simulink library "WBToolboxLibrary"  (R2014b)
settings: Solver=ode45  StartTime=0.0  StopTime=10.0  RelTol=1e-3
undefined symbols (not defined in the file): WBT_modelName, WBT_robotName, WBT_wbiFilename, WBT_wbiList
libraries: simulink x1
(part 1 of 2)
settings Model: Creator=jorhabib  LastModifiedBy=makaveli

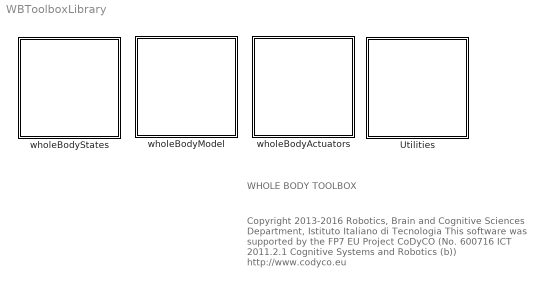
== system WBToolboxLibrary ==
  note: WHOLE BODY TOOLBOX
  note: Copyright  2013-2016 Robotics, Brain and Cognitive Sciences Department, Istituto Italiano di Tecnologia
      | This software was supported by the FP7 EU Project CoDyCO (No. 600716 ICT 2011.2.1 Cognitive Systems and Robotics (b))
      | http://www.codyco.eu
  Utilities : Subsystem
      mask Display: image(imread('utilities.png'))
  wholeBodyActuators : Subsystem
      mask Display: image(imread('wholeBodyActuators.png'),'center')
  wholeBodyModel : Subsystem
      mask Display: image(imread('wholeBodyModel.png'),'center')
  wholeBodyStates : Subsystem
      mask Display: image(imread('wholeBodyStates.png'),'center');

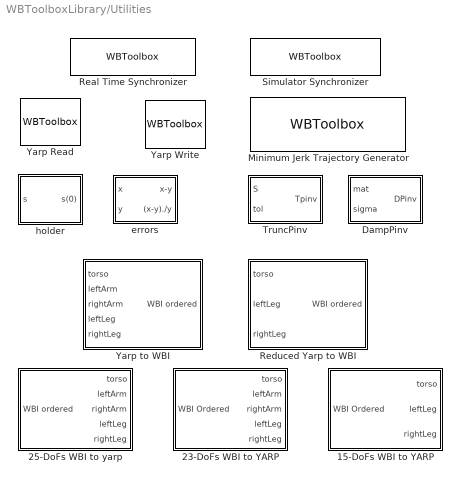
== system WBToolboxLibrary/Utilities ==
  15-DoFs WBI to YARP : Subsystem
      mask help: This is a 23-DoF iCub specific block that swaps first and third joints of the iCub torso from a WBI whole body state reading.
  23-DoFs WBI to YARP : Subsystem
      mask help: This is a 23-DoF iCub specific block that swaps first and third joints of the iCub torso from a WBI whole body state reading.
  25-DoFs WBI to yarp : Subsystem  mask(WBI to YARP){}
      mask help: This is a 25-DOF iCub specific block that swaps first and third joints of the iCub torso from a WBI whole body state reading.
  DampPinv : Subsystem  mask{tol=1e-4}
      mask prompts: tol "Tolerance"
  Minimum Jerk Trajectory Generator : S-Function  FunctionName=WBToolbox  Parameters='MinimumJerkTrajectoryGenerator',sampleTime, settlingTime, firstDerivatives, secondDerivatives, explicitInitialValue, externalSettlingTime  SFunctionDeploymentMode=off  EnableBusSupport=off  mask(Minimum Jerk Trajectory Generator){externalSettlingTime=off, settlingTime=3, sampleTime=0.01, firstDerivatives=on, secondDerivatives=on, explicitInitialValue=off}
      mask prompts: externalSettlingTime "External Settling Time"; settlingTime "Settling Time"; sampleTime "Sample Time"; firstDerivatives "Output First Derivative"; secondDerivatives "Output Second Derivative"; explicitInitialValue "Explicit Initial Value"
      mask help:
      | This block wraps the minJerkTrajGen class from iCub::ctrl::minJerkTrajGen.
      |
      | The Minimum Jerk Trajectory Generator is approximated using a
      | 3rd order LTI dynamical system
      | (for more details see [1]).
      | Position, velocity and acceleration trajectories are computed.
      |  The main advantage with respect to the standard polynomial
      | form is that if the reference value yd changes
      | there is no need to recompute the filter coefficients.
      |
      | [1] Pattacini, U.; Nori, F.; Natale, L.; Metta, G.; Sandini, G., "An experimental evaluation of a novel minimum-jerk cartesian controller for humanoid robots," in Intelligent Robots and Systems (IROS), 2010 IEEE/RSJ International Conference on , vol., no., pp.1668-1674, 18-22 Oct. 2010
      | doi: 10.1109/IROS.2010.5650851
      | URL: http://ieeexplore.ieee.org/stamp/stamp.jsp?tp=&arnumber=5650851&isnumber=5648787
      mask Callback externalSettlingTime:
      | externalSettlingTime = get_param(gcb, 'externalSettlingTime');
      | visibility = get_param(gcb, 'MaskVisibilities');
      | if(strcmp(externalSettlingTime, 'on'))
      |     visibility{2} = 'off';
      | else
      |     visibility{2} = 'on';
      | end
      | set_param(gcb, 'MaskVisibilities',visibility);
      | clear externalSettlingTime
      mask Display:
      | firstDer = get_param(gcb, 'firstDerivatives');
      | secondDer = get_param(gcb, 'secondDerivatives');
      | initialValues = get_param(gcb, 'explicitInitialValue');
      | externalSettlingTimeParam = get_param(gcb, 'externalSettlingTime');
      | 
      | %Inputs
      | portIndex = 2;
      | port_label('input', 1, 'Reference')
      | if(strcmp(initialValues, 'on'))
      |     port_label('input', portIndex, 'Initial Value')
      |     portIndex = portIndex + 1;
      | end
      | 
      | if(strcmp(externalSettlingTimeParam, 'on'))
      |     port_label('input', portIndex, 'Settling Time')
      |     portIndex = portIndex + 1;
      | end
      | 
      | %Outputs
      | port_label('output', 1, 'Signal')
      | secondDerPortIndex = 2;
      | if(strcmp(firstDer, 'on'))
      |     port_label('output', 2, 'First Derivative')
      |     secondDerPortIndex = secondDerPortIndex + 1;
      | end
      | if(strcmp(secondDer, 'on'))
      |     port_label('output', secondDerPortIndex, 'Second Derivative')
      | end
  Real Time Synchronizer : S-Function  FunctionName=WBToolbox  Parameters='RealTimeSynchronizer',period  SFunctionDeploymentMode=off  EnableBusSupport=off  mask(Real Time Synchronizer){period=0.01}
      mask prompts: period "Controller Period (in seconds)"
      mask help:
      | This block slows down the simulation trying to match the period specified
      | as parameter (in seconds).
      | The bigger the period the more probable
      | is that Simulink can remain synched with it.
      mask Display: disp('Real Time Synchronizer')
  Reduced Yarp to WBI : Subsystem  mask(YARP to wbi){}
      mask help:
      | DEPRECATED
      |
      | Please use the explicit 25-DOF or the 23-DOF utility.
      | This block will soon be removed from the Library
      |
      | This is a 25-DOF iCub specific block which swaps the readings of the first and third joint of the torso to comply with WBI order.
  Simulator Synchronizer : S-Function  FunctionName=WBToolbox  Parameters='SimulatorSynchronizer',period, serverPortName, clientPortName  SFunctionDeploymentMode=off  EnableBusSupport=off  mask(Simulator Synchronizer){period=0.01, serverPortName='/clock/rpc', clientPortName='/WBT_synchronizer/rpc:o'}
      mask prompts: period "Controller Period (in seconds)"; serverPortName "Server Port Name"; clientPortName "Client Port Name"
      mask help:
      | This block synchronizes with the external simulation on a simulator
      | (only Gazebo is supported at the moment).
      mask Display: disp('Simulator Synchronizer')
  TruncPinv : Subsystem  mask{tol=1e-4}
      mask prompts: tol "Tolerance"
  Yarp Read : S-Function  FunctionName=WBToolbox  Parameters='YarpRead',portName,signalSize,blocking,timestamp,autoconnect,errorOnConnection  SFunctionDeploymentMode=off  EnableBusSupport=off  mask(YARP Read){portName='/portname', signalSize=1, blocking=off, timestamp=on, autoconnect=on, errorOnConnection=on}
      mask prompts: portName "Source Port Name"; signalSize "Port Size"; blocking "Blocking Read"; timestamp "Read Timestamp"; errorOnConnection "Error on missing connection"
      mask help:
      | This block behaves as the command 'yarp read'.
      | By default it has the option 'Autoconnect' active, which means that the user
      | can only specify the name of the port ('Source Port Name') from which readings are desired,
      | along with the size of the expected data (e.g. 3 when reading the torso state).
      | When the user unchecks 'Autoconnect' 'Opened Port Name' field shows up
      | corresponding to the name of the port the block will create
      | but won't connect to anything.
      | At this point the output will be always zero, until the user connects it
      | to some other port from command line by issuing 'yarp connect [from] [dest]'.
      | In this case an additional output, called 'signal' will be added which will output
      | 1 if the port has received at least one data, or 0 otherwise.
      mask Callback autoconnect:
      | autoconnect_val = get_param(gcb, 'Autoconnect');
      | prompt_string = get_param(gcb, 'MaskPrompts');
      | if(strcmp(autoconnect_val, 'on'))
      |     prompt_string{1} = 'Source Port Name';
      |     set_param(gcb, 'MaskVisibilities',{'on';'on';'on';'on';'on';'on'});
      | else
      |     prompt_string{1} = 'Opened Port Name';
      |     set_param(gcb, 'MaskVisibilities',{'on';'on';'on';'on';'on';'off'});
      | end
      | set_param(gcb, 'MaskPrompts', prompt_string);
      | clear autoconnect_val prompt_string
      mask Display:
      | port_label('output', 1, 'signal');
      | portNumber = 1;
      | if (timestamp)
      |     portNumber = portNumber + 1;
      |     port_label('output', portNumber, 'timestamp');
      | end
      | 
      | if (~autoconnect)
      |     portNumber = portNumber + 1;
      |     port_label('output', portNumber, 'status');
      | end
  Yarp Write : S-Function  FunctionName=WBToolbox  Parameters='YarpWrite',portName,autoconnect,errorOnConnection  SFunctionDeploymentMode=off  EnableBusSupport=off  mask(YARP Write){portName='/portname', autoconnect=off, errorOnConnection=on}
      mask prompts: portName "Opened Port Name"; errorOnConnection "Error on missing connection"
      mask help:
      | This block behaves as the command 'yarp write'.
      |
      | By default this block opens a port names as the "Opened Port Name" parameter
      | and stream the input signal to that port.
      | If the option "Autoconnect" is specified, the first parameter become the
      | name of the target port to which the data will be stramed,
      | e.g. like "yarp write ... /destinationPort"
      mask Callback autoconnect:
      | autoconnect_val = get_param(gcb, 'Autoconnect');
      | prompt_string = get_param(gcb, 'MaskPrompts');
      | if(strcmp(autoconnect_val, 'on'))
      |     prompt_string{1} = 'Destination Port Name';
      |     set_param(gcb, 'MaskVisibilities',{'on';'on';'on'});
      | else
      |     prompt_string{1} = 'Opened Port Name';
      |     set_param(gcb, 'MaskVisibilities',{'on';'on';'off'});
      | end
      | set_param(gcb, 'MaskPrompts', prompt_string);
      | clear autoconnect_val prompt_string
      mask Display: disp('Yarp Write')
  Yarp to WBI : Subsystem  mask(YARP to wbi){}
      mask help:
      | DEPRECATED
      |
      | Please use the explicit 25-DOF or the 23-DOF utility.
      | This block will soon be removed from the Library
      |
      | This is a 25-DOF iCub specific block which swaps the readings of the first and third joint of the torso to comply with WBI order.
  errors : Subsystem  mask(Errors){}
      mask help:
      | Computes two kinds of errors. The first is just the difference between x
      | and y while the second is the ratio (x-y)/y.
  "holder " : Subsystem  mask(Holder){}
      mask help: This block holds the first input value during the simulation.

== system WBToolboxLibrary/wholeBodyActuators ==
  Set LowLevel PIDs : Subsystem  InitFcn=|  mask(Set Low Level PIDs){pidParameters='', pidType=Torque, robotName=WBT_robotName, localName=WBT_modelName, wbiFile=WBT_wbiFilename, wbiList=WBT_wbiList}
      | if ~exist('WBT_robotName','var')
      |     WBT_robotName = '';
      | end
      | if ~exist('WBT_modelName','var')
      |     WBT_modelName = 'WBT_simulink';
      | end
      | if ~exist('WBT_wbiFilename','var')
      |     WBT_wbiFilename = 'yarpWholeBodyInterface.ini';
      | end
      | if ~exist('WBT_wbiList','var')
      |     WBT_wbiList = 'ROBOT_TORQUE_CONTROL_JOINTS';
      | end
      mask prompts: pidParameters "PID parameter"; pidType "PID Type"; robotName "Robot Port Name"; localName "Model Name"; wbiFile "WBI filename"; wbiList "WBI list name"
      mask help:
      | This block sets the low level PID values for the robot actuators.
      |
      | If only one gain file is specified, those gains are loaded at startup.
      | Otherwise an additional port to this block is added which accept an integer
      | representing the index in the list of gains to be loaded (also at runtime)
      |
      | Assuming DoFs is the number of degrees of freedom of the robot,
      | Parameters:
      | - PID Parameter: String specifying either a file containing the PIDs for the
      |                  low level control, or a list of files (in yarp Bottle format).
      |
      | - Robot Port Name: Name of the ports opened by the robot. (e.g. icub).
      |                    Set an empty string ('') to use the name specified in the
      |                    Whole Body Interface configuration file.
      | - Model Name: Prefix name of the ports opened by the underlying Whole Body Interface.
      | - WBI filename: name of the file containing the configuration of the Whole Body Interface
      | - WBI List Name: name of the list of joints used to configure the Whole Body Interface
      mask TypeOptions pidType: Position | Torque
      mask Callback pidType:
      | % Get the mask parameter values. This is a cell
      | %   array of strings.
      | maskStr = get_param(gcb,'pidType');
      | if strcmp(maskStr, 'Position')
      |     set_param(gcb,'BackgroundColor', '[0.5137, 0.8510, 0.6706, 1.0]');
      | elseif strcmp(maskStr, 'Position Direct')
      |     set_param(gcb,'BackgroundColor', '[0.3922, 0.7882, 0.3451, 1.0]');
      | elseif strcmp(maskStr, 'Velocity')
      |     set_param(gcb,'BackgroundColor', '[0.5137, 0.6745, 1.0000, 1.0]');
      | elseif strcmp(maskStr, 'Torque')
      |     set_param(gcb,'BackgroundColor', '[0.8275, 0.5765, 0.6039, 1.0]');
      | end
      | clear  maskStr
      mask Display:
      | pidType = get_param(gcb,'pidType');
      | description = sprintf('Set Low Level\n%s PIDs', pidType);
      | disp(description);
  Set References : Subsystem  InitFcn=|  mask(Set References){controlType=Position, robotName=WBT_robotName, localName=WBT_modelName, wbiFile=WBT_wbiFilename, wbiList=WBT_wbiList}
      | if ~exist('WBT_robotName','var')
      |     WBT_robotName = '';
      | end
      | if ~exist('WBT_modelName','var')
      |     WBT_modelName = 'WBT_simulink';
      | end
      | if ~exist('WBT_wbiFilename','var')
      |     WBT_wbiFilename = 'yarpWholeBodyInterface.ini';
      | end
      | if ~exist('WBT_wbiList','var')
      |     WBT_wbiList = 'ROBOT_TORQUE_CONTROL_JOINTS';
      | end
      mask prompts: controlType "Control Mode"; robotName "Robot Port Name"; localName "Model Name"; wbiFile "WBI filename"; wbiList "WBI list name"
      mask help:
      | This block sets the references for the robot actuators.
      | The type of control mode is specified as a parameter in the block.
      |
      | Assuming DoFs is the number of degrees of freedom of the robot,
      | Input:
      | - References: Vector of size DoFs, representing the references to be sent
      |                 to the robot controlled joints.
      |
      | Parameters:
      | - Control Mode: The control mode. Choose one of the supplied mode.
      |
      | - Robot Port Name: Name of the ports opened by the robot. (e.g. icub).
      |                    Set an empty string ('') to use the name specified in the
      |                    Whole Body Interface configuration file.
      | - Model Name: Prefix name of the ports opened by the underlying Whole Body Interface.
      | - WBI filename: name of the file containing the configuration of the Whole Body Interface
      | - WBI List Name: name of the list of joints used to configure the Whole Body Interface
      mask TypeOptions controlType: Position | Position Direct | Velocity | Torque | Open Loop
      mask Callback controlType:
      | % Get the mask parameter values. This is a cell
      | %   array of strings.
      | maskStr = get_param(gcb,'controlType');
      | if strcmp(maskStr, 'Position')
      |     set_param(gcb,'BackgroundColor', '[0.5137, 0.8510, 0.6706, 1.0]');
      | elseif strcmp(maskStr, 'Position Direct')
      |     set_param(gcb,'BackgroundColor', '[0.3922, 0.7882, 0.3451, 1.0]');
      | elseif strcmp(maskStr, 'Velocity')
      |     set_param(gcb,'BackgroundColor', '[0.5137, 0.6745, 1.0000, 1.0]');
      | elseif strcmp(maskStr, 'Torque')
      |     set_param(gcb,'BackgroundColor', '[0.8275, 0.5765, 0.6039, 1.0]');
      | elseif strcmp(maskStr, 'Open Loop')
      |     set_param(gcb,'BackgroundColor', '[0.98, 0.98, 0.98, 1.0]');
      | end
      | clear  maskStr
      mask Display:
      | disp(get_param(gcb,'controlType'))
      | %port_label('input',1,'References')

== system WBToolboxLibrary/wholeBodyModel ==
  Dynamics : Subsystem
      mask Display: image(imread('Dynamics.png'))
  Jacobians : Subsystem
      mask Display: image(imread('jacobian.png'))
  Kinematics : Subsystem
      mask Display: image(imread('forwardKinematics.png'))

== system WBToolboxLibrary/wholeBodyStates ==
  Get Estimate : Subsystem  InitFcn=|  mask(Get Estimate){estimateType=Joints Position, robotName=WBT_robotName, localName=WBT_modelName, wbiFile=WBT_wbiFilename, wbiList=WBT_wbiList}
      | if ~exist('WBT_robotName','var')
      |     WBT_robotName = '';
      | end
      | if ~exist('WBT_modelName','var')
      |     WBT_modelName = 'WBT_simulink';
      | end
      | if ~exist('WBT_wbiFilename','var')
      |     WBT_wbiFilename = 'yarpWholeBodyInterface.ini';
      | end
      | if ~exist('WBT_wbiList','var')
      |     WBT_wbiList = 'ROBOT_TORQUE_CONTROL_JOINTS';
      | end
      mask prompts: estimateType "Estimate Type"; robotName "Robot Port Name"; localName "Model Name"; wbiFile "WBI filename"; wbiList "WBI list name"
      mask help:
      | This block get the estimate of the specified type
      |
      | Assuming DoFs is the number of degrees of freedom of the robot,
      | Output:
      | - References: Vector of size DoFs, representing the estimate requested.
      |
      | Parameters:
      | - Control Mode: The control mode. Choose one of the supplied mode.
      |
      | - Robot Port Name: Name of the ports opened by the robot. (e.g. icub).
      |                    Set an empty string ('') to use the name specified in the
      |                    Whole Body Interface configuration file.
      | - Model Name: Prefix name of the ports opened by the underlying Whole Body Interface.
      | - WBI filename: name of the file containing the configuration of the Whole Body Interface
      | - WBI List Name: name of the list of joints used to configure the Whole Body Interface
      mask TypeOptions estimateType: Joints Position | Joints Velocity | Joints Acceleration | Joints Torque
      mask Callback estimateType:
      | % Get the mask parameter values. This is a cell
      | %   array of strings.
      | 
      | maskStr = get_param(gcb,'estimateType');
      | if strcmp(maskStr, 'Joints Position')
      |     set_param(gcb,'BackgroundColor', '[0.5137, 0.8510, 0.6706, 1.0]');
      | elseif strcmp(maskStr, 'Joints Velocity')
      |     set_param(gcb,'BackgroundColor', '[0.5137, 0.6745, 1.0000, 1.0]');
      | elseif strcmp(maskStr, 'Joints Acceleration')
      |     set_param(gcb,'BackgroundColor', '[0.9255, 0.8706, 0.1333, 1.0]');
      | elseif strcmp(maskStr, 'Joints Torque')
      |     set_param(gcb,'BackgroundColor', '[0.8275, 0.5765, 0.6039, 1.0]');
      | end
      | clear  maskStr
      mask Display:
      | %disp(get_param(gcb,'estimateType'))
      | port_label('output',1,get_param(gcb,'estimateType'))
  Get Limits : Subsystem  InitFcn=|  mask(Get Estimate){limitsType=Position, robotName=WBT_robotName, localName=WBT_modelName, wbiFile=WBT_wbiFilename, wbiList=WBT_wbiList}
      | if ~exist('WBT_robotName','var')
      |     WBT_robotName = '';
      | end
      | if ~exist('WBT_modelName','var')
      |     WBT_modelName = 'WBT_simulink';
      | end
      | if ~exist('WBT_wbiFilename','var')
      |     WBT_wbiFilename = 'yarpWholeBodyInterface.ini';
      | end
      | if ~exist('WBT_wbiList','var')
      |     WBT_wbiList = 'ROBOT_TORQUE_CONTROL_JOINTS';
      | end
      mask prompts: limitsType "Limits Type"; robotName "Robot Port Name"; localName "Model Name"; wbiFile "WBI filename"; wbiList "WBI list name"
      mask help:
      | This block get the estimate of the specified type
      |
      | Assuming DoFs is the number of degrees of freedom of the robot,
      | Output:
      | - References: Vector of size DoFs, representing the estimate requested.
      |
      | Parameters:
      | - Control Mode: The control mode. Choose one of the supplied mode.
      |
      | - Robot Port Name: Name of the ports opened by the robot. (e.g. icub).
      |                    Set an empty string ('') to use the name specified in the
      |                    Whole Body Interface configuration file.
      | - Model Name: Prefix name of the ports opened by the underlying Whole Body Interface.
      | - WBI filename: name of the file containing the configuration of the Whole Body Interface
      | - WBI List Name: name of the list of joints used to configure the Whole Body Interface
      mask TypeOptions limitsType: Position
      mask Callback limitsType:
      | % Get the mask parameter values. This is a cell
      | %   array of strings.
      | 
      | maskStr = get_param(gcb,'limitsType');
      | if strcmp(maskStr, 'Joints Position')
      |     set_param(gcb,'BackgroundColor', '[0.5137, 0.8510, 0.6706, 1.0]');
      | elseif strcmp(maskStr, 'Joints Velocity')
      |     set_param(gcb,'BackgroundColor', '[0.5137, 0.6745, 1.0000, 1.0]');
      | elseif strcmp(maskStr, 'Joints Acceleration')
      |     set_param(gcb,'BackgroundColor', '[0.9255, 0.8706, 0.1333, 1.0]');
      | elseif strcmp(maskStr, 'Joints Torque')
      |     set_param(gcb,'BackgroundColor', '[0.8275, 0.5765, 0.6039, 1.0]');
      | end
      | clear  maskStr
      mask Display:
      | disp(get_param(gcb,'limitsType'))
      | port_label('output',1,'Min')
      | port_label('output',2,'Max')

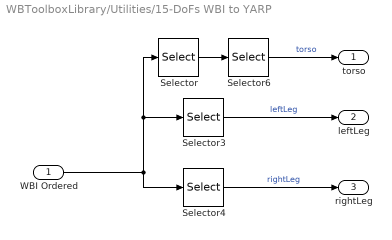
== system WBToolboxLibrary/Utilities/15-DoFs WBI to YARP ==
  WBI Ordered : Inport
  Selector : Selector  InputPortWidth=ROBOT_DOF  IndexOptions=Index vector (dialog)  Indices=[1:3]  OutputSizes=1
  Selector3 : Selector  InputPortWidth=ROBOT_DOF  IndexOptions=Index vector (dialog)  Indices=[12:17]  OutputSizes=1
  Selector4 : Selector  InputPortWidth=ROBOT_DOF  IndexOptions=Index vector (dialog)  Indices=[18:23]  OutputSizes=1
  Selector6 : Selector  InputPortWidth=3  IndexOptions=Index vector (dialog)  Indices=[3 2 1]  OutputSizes=1
  torso : Outport
  leftLeg : Outport  Port=2
  rightLeg : Outport  Port=3
  wires:
  Selector/1 -> Selector6/1
  Selector6/1 -> torso/1  "torso"
  WBI Ordered/1 -> Selector3/1, Selector/1, Selector4/1
  Selector3/1 -> leftLeg/1  "leftLeg"
  Selector4/1 -> rightLeg/1  "rightLeg"

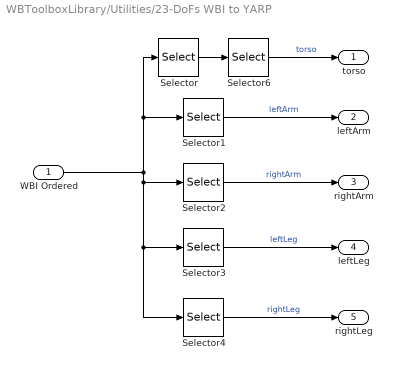
== system WBToolboxLibrary/Utilities/23-DoFs WBI to YARP ==
  WBI Ordered : Inport
  Selector : Selector  InputPortWidth=ROBOT_DOF  IndexOptions=Index vector (dialog)  Indices=[1:3]  OutputSizes=1
  Selector1 : Selector  InputPortWidth=ROBOT_DOF  IndexOptions=Index vector (dialog)  Indices=[4:7]  OutputSizes=1
  Selector2 : Selector  InputPortWidth=ROBOT_DOF  IndexOptions=Index vector (dialog)  Indices=[8:11]  OutputSizes=1
  Selector3 : Selector  InputPortWidth=ROBOT_DOF  IndexOptions=Index vector (dialog)  Indices=[12:17]  OutputSizes=1
  Selector4 : Selector  InputPortWidth=ROBOT_DOF  IndexOptions=Index vector (dialog)  Indices=[18:23]  OutputSizes=1
  Selector6 : Selector  InputPortWidth=3  IndexOptions=Index vector (dialog)  Indices=[3 2 1]  OutputSizes=1
  torso : Outport
  leftArm : Outport  Port=2
  rightArm : Outport  Port=3
  leftLeg : Outport  Port=4
  rightLeg : Outport  Port=5
  wires:
  Selector/1 -> Selector6/1
  Selector6/1 -> torso/1  "torso"
  WBI Ordered/1 -> Selector/1, Selector1/1, Selector2/1, Selector4/1, Selector3/1
  Selector1/1 -> leftArm/1  "leftArm"
  Selector2/1 -> rightArm/1  "rightArm"
  Selector3/1 -> leftLeg/1  "leftLeg"
  Selector4/1 -> rightLeg/1  "rightLeg"

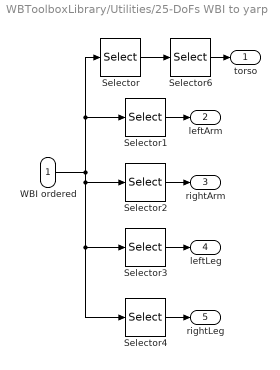
== system WBToolboxLibrary/Utilities/25-DoFs WBI to yarp ==
  WBI ordered : Inport
  Selector : Selector  InputPortWidth=ROBOT_DOF  IndexOptions=Index vector (dialog)  Indices=[1:3]  OutputSizes=1
  Selector1 : Selector  InputPortWidth=ROBOT_DOF  IndexOptions=Index vector (dialog)  Indices=[4:8]  OutputSizes=1
  Selector2 : Selector  InputPortWidth=ROBOT_DOF  IndexOptions=Index vector (dialog)  Indices=[9:13]  OutputSizes=1
  Selector3 : Selector  InputPortWidth=ROBOT_DOF  IndexOptions=Index vector (dialog)  Indices=[14:19]  OutputSizes=1
  Selector4 : Selector  InputPortWidth=ROBOT_DOF  IndexOptions=Index vector (dialog)  Indices=[20:25]  OutputSizes=1
  Selector6 : Selector  InputPortWidth=3  IndexOptions=Index vector (dialog)  Indices=[3 2 1]  OutputSizes=1
  torso : Outport
  leftArm : Outport  Port=2
  rightArm : Outport  Port=3
  leftLeg : Outport  Port=4
  rightLeg : Outport  Port=5
  wires:
  Selector1/1 -> leftArm/1
  Selector2/1 -> rightArm/1
  Selector3/1 -> leftLeg/1
  Selector4/1 -> rightLeg/1
  WBI ordered/1 -> Selector/1, Selector1/1, Selector2/1, Selector4/1, Selector3/1
  Selector/1 -> Selector6/1
  Selector6/1 -> torso/1

== system WBToolboxLibrary/Utilities/DampPinv ==
  mat : Inport
  sigma : Inport  Port=2
  Damped Pseudo Inverse : MATLAB Function  TreatAsAtomicUnit=on
      settings: PermitHierarchicalResolution=ParametersOnly
  DPinv : Outport
  wires:
  sigma/1 -> Damped Pseudo Inverse/2(sigma)
  Damped Pseudo Inverse/1(DPinv) -> DPinv/1
  mat/1 -> Damped Pseudo Inverse/1(mat)

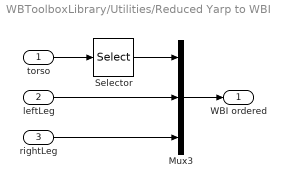
== system WBToolboxLibrary/Utilities/Reduced Yarp to WBI ==
  torso : Inport
  leftLeg : Inport  Port=2
  rightLeg : Inport  Port=3
  Mux3 : Mux  Inputs=3
  Selector : Selector  InputPortWidth=3  IndexOptions=Index vector (dialog)  Indices=[3 2 1]  OutputSizes=1
  WBI ordered : Outport
  wires:
  Selector/1 -> Mux3/1
  torso/1 -> Selector/1
  Mux3/1 -> WBI ordered/1
  leftLeg/1 -> Mux3/2
  rightLeg/1 -> Mux3/3

== system WBToolboxLibrary/Utilities/TruncPinv ==
  S : Inport
  tol : Inport  Port=2
  Truncated PseudoInverse : MATLAB Function  TreatAsAtomicUnit=on
      settings: PermitHierarchicalResolution=ParametersOnly
  Tpinv : Outport
  wires:
  S/1 -> Truncated PseudoInverse/1(mat)
  Truncated PseudoInverse/1(TPinv) -> Tpinv/1
  tol/1 -> Truncated PseudoInverse/2(tol)

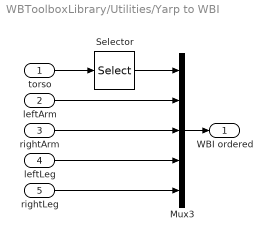
== system WBToolboxLibrary/Utilities/Yarp to WBI ==
  torso : Inport
  leftArm : Inport  Port=2
  rightArm : Inport  Port=3
  leftLeg : Inport  Port=4
  rightLeg : Inport  Port=5
  Mux3 : Mux  Inputs=5
  Selector : Selector  InputPortWidth=3  IndexOptions=Index vector (dialog)  Indices=[3 2 1]  OutputSizes=1
  WBI ordered : Outport
  wires:
  Selector/1 -> Mux3/1
  torso/1 -> Selector/1
  leftArm/1 -> Mux3/2
  rightArm/1 -> Mux3/3
  Mux3/1 -> WBI ordered/1
  leftLeg/1 -> Mux3/4
  rightLeg/1 -> Mux3/5

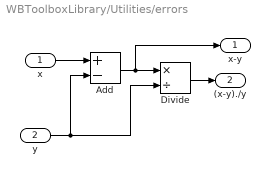
== system WBToolboxLibrary/Utilities/errors ==
  x : Inport
  y : Inport  Port=2
  Add : Sum  Inputs=+-
  Divide : Product  Inputs=*/
  x-y : Outport
  (x-y)./y : Outport  Port=2
  wires:
  Add/1 -> Divide/1, x-y/1
  x/1 -> Add/1
  y/1 -> Add/2, Divide/2
  Divide/1 -> (x-y)./y/1

== system WBToolboxLibrary/Utilities/holder  ==
  s : Inport
  Clock : Clock
  Compare To Constant : simulink/Logic and Bit Operations/Compare To Constant  relop===  const=0  OutDataTypeStr=boolean
  MATLAB Function : MATLAB Function  TreatAsAtomicUnit=on
      settings: PermitHierarchicalResolution=ParametersOnly
  s(0) : Outport
  wires:
  Clock/1 -> Compare To Constant/1
  MATLAB Function/1(s0) -> s(0)/1
  s/1 -> MATLAB Function/1(s)
  Compare To Constant/1 -> MATLAB Function/2(unused)

== system WBToolboxLibrary/wholeBodyActuators/Set LowLevel PIDs ==
  S-Function : S-Function  FunctionName=WBToolbox  Parameters='SetLowLevelPID',robotName,localName,wbiFile,wbiList,pidParameters,pidType  SFunctionDeploymentMode=off  EnableBusSupport=off

== system WBToolboxLibrary/wholeBodyActuators/Set References ==
  References : Inport
  S-Function : S-Function  FunctionName=WBToolbox  Parameters='SetReferences',robotName,localName,wbiFile,wbiList,controlType  SFunctionDeploymentMode=off  EnableBusSupport=off
  wires:
  References/1 -> S-Function/1

== system WBToolboxLibrary/wholeBodyModel/Dynamics ==
  Centroidal Momentum : Subsystem  InitFcn=|  mask(Centroidal Momentum){robotName=WBT_robotName, localName=WBT_modelName, wbiFile=WBT_wbiFilename, wbiList=WBT_wbiList}
      | if ~exist('WBT_robotName','var')
      |     WBT_robotName = '';
      | end
      | if ~exist('WBT_modelName','var')
      |     WBT_modelName = 'WBT_simulink';
      | end
      | if ~exist('WBT_wbiFilename','var')
      |     WBT_wbiFilename = 'yarpWholeBodyInterface.ini';
      | end
      | if ~exist('WBT_wbiList','var')
      |     WBT_wbiList = 'ROBOT_TORQUE_CONTROL_JOINTS';
      | end
      mask prompts: robotName "Robot Port Name"; localName "Model Name"; wbiFile "WBI filename"; wbiList "WBI list name"
      mask help:
      | This block computed the 6 element centroidal momentum, as defined in:
      | "Centroidal dynamics of a humanoid robot" - DE Orin, A Goswami, SH Lee -
      | Autonomous Robots 35 (2-3), 161-176
      |
      | Assuming DoFs is the number of degrees of freedom of the robot,
      | Input:
      | - Base pose: 4x4 matrix representing the homogenous transformation between
      |              the base frame and the world frame.
      | - Joint configuration: Vector of size DoFs, representing the configuration
      |                        of the joints.
      | - Base velocity: Vector of size 6 representing the linear and angular velocity
      |                  of the base frame.
      | - Joints velocity: Vector of size DoFs, representing the velocity
      |                    of the joints.
      |
      | Output:
      | - Centroidal Momentum: 6-element vector containg the centroidal momentum
      |                 (3 value for linear momentum and 3 for angular momentum)
      |
      | Parameters:
      | - Robot Port Name: Name of the ports opened by the robot. (e.g. icub).
      |                    Set an empty string ('') to use the name specified in the
      |                    Whole Body Interface configuration file.
      | - Model Name: Prefix name of the ports opened by the underlying Whole Body Interface.
      | - WBI filename: name of the file containing the configuration of the Whole Body Interface
      | - WBI List Name: name of the list of joints used to configure the Whole Body Interface
  Get Bias Forces : Subsystem  InitFcn=|  mask(Get Generalized Bias Forces){robotName=WBT_robotName, localName=WBT_modelName, wbiFile=WBT_wbiFilename, wbiList=WBT_wbiList, explicitGravity=off}
      | if ~exist('WBT_robotName','var')
      |     WBT_robotName = '';
      | end
      | if ~exist('WBT_modelName','var')
      |     WBT_modelName = 'WBT_simulink';
      | end
      | if ~exist('WBT_wbiFilename','var')
      |     WBT_wbiFilename = 'yarpWholeBodyInterface.ini';
      | end
      | if ~exist('WBT_wbiList','var')
      |     WBT_wbiList = 'ROBOT_TORQUE_CONTROL_JOINTS';
      | end
      mask prompts: robotName "Robot Port Name"; localName "Model Name"; wbiFile "WBI filename"; wbiList "WBI list name"; explicitGravity "Explicit Gravity"
      mask help:
      | This block retrieves the generalied bias forces of the robot.
      |
      | Parameter:
      | - Explicit Gravity. If True, an additional port (explicit Gravity) is added.
      |                     Otherwise the vector [0; 0; -9.81] is used.
      | Assuming DoFs is the number of degrees of freedom of the robot,
      | Input:
      | - Base pose: 4x4 matrix representing the homogenous transformation between
      |             the base frame and the world frame.
      | - Joint configuration: Vector of size DoFs, representing the configuration
      |                     of the joints.
      | - Base velocity: Vector of size 6 representing the linear and angular velocity
      |                  of the base frame.
      | - Joints velocity: Vector of size DoFs, representing the velocity of the joints.
      |
      | Output:
      | - Bias Forces: a Dofs + 6 vector representing the generalized bias forces
      |             of the robot
      |
      | Parameters:
      | - Robot Port Name: Name of the ports opened by the robot. (e.g. icub).
      |                    Set an empty string ('') to use the name specified in the
      |                     Whole Body Interface configuration file.
      | - Model Name: Prefix name of the ports opened by the underlying Whole Body Interface.
      | - WBI filename: name of the file containing the configuration of the Whole Body Interface
      | - WBI List Name: name of the list of joints used to configure the Whole Body Interface
      mask init:
      | gravityInput = find_system(gcb, ...
      | 'LookUnderMasks', 'on', ...
      | 'FollowLinks', 'on', ...
      | 'Name', 'Gravity');
      | 
      | if explicitGravity
      |     if isempty(gravityInput)
      |         Simulink.Block.eval([gcb,'/S-Function']);
      |         add_block('built-in/Inport',[gcb,'/Gravity']);
      |         add_line(gcb','Gravity/1','S-Function/7', 'autorouting','on');
      |     end
      | else
      |     if ~isempty(gravityInput)
      |         delete_line(gcb','Gravity/1','S-Function/7');
      |         delete_block(gravityInput);
      |         Simulink.Block.eval([gcb,'/S-Function']);
      |     end
      | end
  Get Gravity Forces : Subsystem  InitFcn=|  mask(Gravity bias){robotName=WBT_robotName, localName=WBT_modelName, wbiFile=WBT_wbiFilename, wbiList=WBT_wbiList, explicitGravity=off}
      | if ~exist('WBT_robotName','var')
      |     WBT_robotName = '';
      | end
      | if ~exist('WBT_modelName','var')
      |     WBT_modelName = 'WBT_simulink';
      | end
      | if ~exist('WBT_wbiFilename','var')
      |     WBT_wbiFilename = 'yarpWholeBodyInterface.ini';
      | end
      | if ~exist('WBT_wbiList','var')
      |     WBT_wbiList = 'ROBOT_TORQUE_CONTROL_JOINTS';
      | end
      mask prompts: robotName "Robot Port Name"; localName "Model Name"; wbiFile "WBI filename"; wbiList "WBI list name"; explicitGravity "Explicit Gravity"
      mask help:
      | This block compute the generalized bias forces due to the gravity
      |
      | Parameter:
      | - Explicit Gravity. If True, an additional port (explicit Gravity) is added.
      |                     Otherwise the vector [0; 0; -9.81] is used.
      |
      | Assuming DoFs is the number of degrees of freedom of the robot,
      | Input:
      | - Base pose: 4x4 matrix representing the homogenous transformation between
      |              the base frame and the world frame.
      | - Joint configuration: Vector of size DoFs, representing the configuration
      |                        of the joints.
      |
      | Output:
      | - Gravity: a Dofs + 6 vector representing the torques due to the gravity.
      |
      | Parameters:
      | - Robot Port Name: Name of the ports opened by the robot. (e.g. icub).
      |                    Set an empty string ('') to use the name specified in the
      |                    Whole Body Interface configuration file.
      | - Model Name: Prefix name of the ports opened by the underlying Whole Body Interface.
      | - WBI filename: name of the file containing the configuration of the Whole Body Interface
      | - WBI List Name: name of the list of joints used to configure the Whole Body Interface
      mask init: same as WBToolboxLibrary/wholeBodyModel/Dynamics/Get Bias Forces
  Inverse Dynamics : S-Function  FunctionName=WBToolbox  Parameters='InverseDynamics',robotName,localName,wbiFile,wbiList,explicitGravity  SFunctionDeploymentMode=off  EnableBusSupport=off  mask(Inverse Dynamics){robotName=WBT_robotName, localName=WBT_modelName, wbiFile=WBT_wbiFilename, wbiList=WBT_wbiList, explicitGravity=off}
      mask prompts: robotName "Robot Port Name"; localName "Model Name"; wbiFile "WBI filename"; wbiList "WBI list name"; explicitGravity "Explicit Gravity"
      mask help:
      | This block compute the inverse dynamics of the robot.
      |
      | Parameter:
      | - Explicit Gravity. If True, an additional port (explicit Gravity) is added.
      |                     Otherwise the vector [0; 0; -9.81] is used.
      |
      | Assuming DoFs is the number of degrees of freedom of the robot,
      | Input:
      | - Base pose: 4x4 matrix representing the homogenous transformation between
      |              the base frame and the world frame.
      | - Joint configuration: Vector of size DoFs, representing the configuration
      |                        of the joints.
      | - Base velocity: Vector of size 6 representing the linear and angular velocity
      |                  of the base frame.
      | - Joints velocity: Vector of size DoFs, representing the velocity
      |                    of the joints.
      | - Base acceleration: Vector of size 6 representing the linear and angular acceleration
      |                  of the base frame.
      | - Joints acceleration: Vector of size DoFs, representing the acceleration
      |                    of the joints.
      | - Gravity: Vector of size 3, denoting the acceleration vector w.r.t. the world frame.
      |
      |
      | Output:
      | - Torques: a Dofs + 6 vector representing the corresponding torques required
      |            to achive the desired accelerations given the robot state
      |
      | Parameters:
      | - Robot Port Name: Name of the ports opened by the robot. (e.g. icub).
      |                    Set an empty string ('') to use the name specified in the
      |                    Whole Body Interface configuration file.
      | - Model Name: Prefix name of the ports opened by the underlying Whole Body Interface.
      | - WBI filename: name of the file containing the configuration of the Whole Body Interface
      | - WBI List Name: name of the list of joints used to configure the Whole Body Interface
      mask Display:
      | port_label('output', 1, 'Torques')
      | 
      | port_label('input', 1, 'Base pose')
      | port_label('input', 2, 'Joints configuration')
      | port_label('input', 3, 'Base velocity')
      | port_label('input', 4, 'Joints velocity')
      | port_label('input', 5, 'Base acceleration')
      | port_label('input', 6, 'Joints acceleration')
      | 
      | 
      | gravity = get_param(gcb, 'explicitGravity');
      | if(strcmp(gravity, 'on'))
      |     port_label('input', 7, 'Gravity')
      | end
  Mass Matrix : Subsystem  InitFcn=|  mask(Mass Matrix){robotName=WBT_robotName, localName=WBT_modelName, wbiFile=WBT_wbiFilename, wbiList=WBT_wbiList}
      | if ~exist('WBT_robotName','var')
      |     WBT_robotName = '';
      | end
      | if ~exist('WBT_modelName','var')
      |     WBT_modelName = 'WBT_simulink';
      | end
      | if ~exist('WBT_wbiFilename','var')
      |     WBT_wbiFilename = 'yarpWholeBodyInterface.ini';
      | end
      | if ~exist('WBT_wbiList','var')
      |     WBT_wbiList = 'ROBOT_TORQUE_CONTROL_JOINTS';
      | end
      mask prompts: robotName "Robot Port Name"; localName "Model Name"; wbiFile "WBI filename"; wbiList "WBI list name"
      mask help:
      | This block retrieves the robot mass matrix.
      |
      | Assuming DoFs is the number of degrees of freedom of the robot,
      | Input:
      | - Base pose: 4x4 matrix representing the homogenous transformation between
      |              the base frame and the world frame.
      | - Joint configuration: Vector of size DoFs, representing the configuration
      |                        of the joints.
      |
      | Output:
      | - Mass Matrix: a (Dofs + 6) x (Dofs + 6) matrix representing the mass matrix
      |                of the robot
      |
      | Parameters:
      | - Robot Port Name: Name of the ports opened by the robot. (e.g. icub).
      |                    Set an empty string ('') to use the name specified in the
      |                    Whole Body Interface configuration file.
      | - Model Name: Prefix name of the ports opened by the underlying Whole Body Interface.
      | - WBI filename: name of the file containing the configuration of the Whole Body Interface
      | - WBI List Name: name of the list of joints used to configure the Whole Body Interface

== system WBToolboxLibrary/wholeBodyModel/Jacobians ==
  DotJ Nu : Subsystem  InitFcn=|  mask(DotJ Nu){frameName='frame', robotName=WBT_robotName, localName=WBT_modelName, wbiFile=WBT_wbiFilename, wbiList=WBT_wbiList}
      | if ~exist('WBT_robotName','var')
      |     WBT_robotName = '';
      | end
      | if ~exist('WBT_modelName','var')
      |     WBT_modelName = 'WBT_simulink';
      | end
      | if ~exist('WBT_wbiFilename','var')
      |     WBT_wbiFilename = 'yarpWholeBodyInterface.ini';
      | end
      | if ~exist('WBT_wbiList','var')
      |     WBT_wbiList = 'ROBOT_TORQUE_CONTROL_JOINTS';
      | end
      mask prompts: frameName "Frame name"; robotName "Robot Port Name"; localName "Model Name"; wbiFile "WBI filename"; wbiList "WBI list name"
      mask help:
      | This block computes the product between the time derivative of the
      |          Jacobian of the specified frame and the state (base and joints)
      |         velocity vector.
      |
      | Assuming DoFs is the number of degrees of freedom of the robot,
      | Input:
      | - Base pose: 4x4 matrix representing the homogenous transformation between
      |              the the base frame and the world frame.
      | - Joint configuration: Vector of size DoFs, representing the configuration
      |                        of the joints.
      | - Base velocity: Vector of size 6 representing the linear and angular velocity
      |                  of the base frame.
      | - Joints velocity: Vector of size DoFs, representing the velocity
      |                    of the joints.
      |
      | Output:
      | - dotJ nu: a 6-d vector representing the product between the time derivative of the
      |          Jacobian of the specified frame and the state velocity vector
      |
      | Parameters:
      | - Frame name: the name of the frame. It should be specified in the URDF model.
      |
      | - Robot Port Name: Name of the ports opened by the robot. (e.g. icub).
      |                    Set an empty string ('') to use the name specified in the
      |                    Whole Body Interface configuration file.
      | - Model Name: Prefix name of the ports opened by the underlying Whole Body Interface.
      | - WBI filename: name of the file containing the configuration of the Whole Body Interface
      | - WBI List Name: name of the list of joints used to configure the Whole Body Interface
      mask Display:
      | escapedFrameName = strrep(frameName, '_', '\_');
      | port_label('output', 1, strcat('dot J_{',escapedFrameName,'} \nu'), 'texmode','on')
      | 
      | port_label('input', 1, '{}^{world} H_{base}', 'texmode','on')
      | port_label('input', 2, 'Joint configuration')
      | port_label('input', 3, 'Base velocity')
      | port_label('input', 4, 'Joint velocity')
      | 
      | clear escapedFrameName;
  Jacobian : Subsystem  InitFcn=|  mask(Jacobian){frameName='frame', robotName=WBT_robotName, localName=WBT_modelName, wbiFile=WBT_wbiFilename, wbiList=WBT_wbiList}
      | if ~exist('WBT_robotName','var')
      |     WBT_robotName = '';
      | end
      | if ~exist('WBT_modelName','var')
      |     WBT_modelName = 'WBT_simulink';
      | end
      | if ~exist('WBT_wbiFilename','var')
      |     WBT_wbiFilename = 'yarpWholeBodyInterface.ini';
      | end
      | if ~exist('WBT_wbiList','var')
      |     WBT_wbiList = 'ROBOT_TORQUE_CONTROL_JOINTS';
      | end
      mask prompts: frameName "Frame name"; robotName "Robot Port Name"; localName "Model Name"; wbiFile "WBI filename"; wbiList "WBI list name"
      mask help:
      | This block retrieves the Jacobian of the specified frame.
      |
      | Assuming DoFs is the number of degrees of freedom of the robot,
      | Input:
      | - Base pose: 4x4 matrix representing the homogenous transformation between
      |              the the base frame and the world frame.
      | - Joint configuration: Vector of size DoFs, representing the configuration
      |                        of the joints.
      |
      | Output:
      | - Jacobian: a 6x6+dofs matrix representing the Jacobian of
      |              the specified frame written in the world frame.
      |
      | Parameters:
      | - Frame name: the name of the frame. It should be specified in the URDF model.
      |
      | - Robot Port Name: Name of the ports opened by the robot. (e.g. icub).
      |                    Set an empty string ('') to use the name specified in the
      |                    Whole Body Interface configuration file.
      | - Model Name: Prefix name of the ports opened by the underlying Whole Body Interface.
      | - WBI filename: name of the file containing the configuration of the Whole Body Interface
      | - WBI List Name: name of the list of joints used to configure the Whole Body Interface
      mask Display:
      | escapedFrameName = strrep(frameName, '_', '\_');
      | port_label('output', 1, strcat('{}^{world} J_{',escapedFrameName,'}'), 'texmode','on')
      | 
      | port_label('input', 1, '{}^{world} H_{base}', 'texmode','on')
      | port_label('input', 2, 'Joint configuration')
      | 
      | clear escapedFrameName;

== system WBToolboxLibrary/wholeBodyModel/Kinematics ==
  Forward Kinematics : Subsystem  InitFcn=|  mask(Forward Kinematics){frameName='frame', robotName=WBT_robotName, localName=WBT_modelName, wbiFile=WBT_wbiFilename, wbiList=WBT_wbiList}
      | if ~exist('WBT_robotName','var')
      |     WBT_robotName = '';
      | end
      | if ~exist('WBT_modelName','var')
      |     WBT_modelName = 'WBT_simulink';
      | end
      | if ~exist('WBT_wbiFilename','var')
      |     WBT_wbiFilename = 'yarpWholeBodyInterface.ini';
      | end
      | if ~exist('WBT_wbiList','var')
      |     WBT_wbiList = 'ROBOT_TORQUE_CONTROL_JOINTS';
      | end
      mask prompts: frameName "Frame name"; robotName "Robot Port Name"; localName "Model Name"; wbiFile "WBI filename"; wbiList "WBI list name"
      mask help:
      | This block retrieves the forward kinematics of the specified frame.
      |
      | Assuming DoFs is the number of degrees of freedom of the robot,
      | Input:
      | - Base pose: 4x4 matrix representing the homogenous transformation between
      |              the the base frame and the world frame.
      | - Joint configuration: Vector of size DoFs, representing the configuration
      |                        of the joints.
      |
      | Output:
      | - Forward Kinematics: a 4x4 matrix representing the homogenous transformation between
      |              the specified frame and the world frame.
      |
      | Parameters:
      | - Frame name: the name of the frame. It should be specified in the URDF model.
      |
      | - Robot Port Name: Name of the ports opened by the robot. (e.g. icub).
      |                    Set an empty string ('') to use the name specified in the
      |                    Whole Body Interface configuration file.
      | - Model Name: Prefix name of the ports opened by the underlying Whole Body Interface.
      | - WBI filename: name of the file containing the configuration of the Whole Body Interface
      | - WBI List Name: name of the list of joints used to configure the Whole Body Interface
      mask Display:
      | escapedFrameName = strrep(frameName, '_', '\_');
      | port_label('output', 1, strcat('{}^{world} H_{',escapedFrameName,'}'), 'texmode','on')
      | 
      | port_label('input', 1, '{}^{world} H_{base}', 'texmode','on')
      | port_label('input', 2, 'Joint configuration')
      | 
      | clear escapedFrameName;
  Inverse Kinematics : Subsystem  InitFcn=|  mask(Forward Kinematics){robotPart=left, optOption=Full Constraint (Position and Orientation), robotName=WBT_robotName, localName=WBT_modelName, wbiFile=WBT_wbiFilename, wbiList=WBT_wbiList}
      | if ~exist('WBT_robotName','var')
      |     WBT_robotName = '';
      | end
      | if ~exist('WBT_modelName','var')
      |     WBT_modelName = 'WBT_simulink';
      | end
      | if ~exist('WBT_wbiFilename','var')
      |     WBT_wbiFilename = 'yarpWholeBodyInterface.ini';
      | end
      | if ~exist('WBT_wbiList','var')
      |     WBT_wbiList = 'ROBOT_TORQUE_CONTROL_JOINTS';
      | end
      mask prompts: robotPart "Robot Part"; optOption "Optimization Option"; robotName "Robot Port Name"; localName "Model Name"; wbiFile "WBI filename"; wbiList "WBI list name"
      mask help:
      | This block retrieves the forward kinematics of the specified frame.
      |
      | Assuming DoFs is the number of degrees of freedom of the robot,
      | Input:
      | - Base pose: 4x4 matrix representing the homogenous transformation between
      |              the the base frame and the world frame.
      | - Joint configuration: Vector of size DoFs, representing the configuration
      |                        of the joints.
      |
      | Output:
      | - Forward Kinematics: a 4x4 matrix representing the homogenous transformation between
      |              the specified frame and the world frame.
      |
      | Parameters:
      | - Frame name: the name of the frame. It should be specified in the URDF model.
      |
      | - Robot Port Name: Name of the ports opened by the robot. (e.g. icub).
      |                    Set an empty string ('') to use the name specified in the
      |                    Whole Body Interface configuration file.
      | - Model Name: Prefix name of the ports opened by the underlying Whole Body Interface.
      | - WBI filename: name of the file containing the configuration of the Whole Body Interface
      | - WBI List Name: name of the list of joints used to configure the Whole Body Interface
      mask TypeOptions robotPart: left | right
      mask TypeOptions optOption: Full Constraint (Position and Orientation) | Position only constraint
      mask Display:
      | %escapedFrameName = strrep(frameName, '_', '\_');
      | %port_label('output', 1, strcat('{}^{world} H_{',escapedFrameName,'}'), 'texmode','on')
      | 
      | %port_label('input', 1, '{}^{world} H_{base}', 'texmode','on')
      | %port_label('input', 2, 'Joint configuration')
      | 
      | %clear escapedFrameName;
      | 
      | 
      | if strcmp(robotPart, 'left')
      |     prefix = 'l';
      | else
      |     prefix = 'r';
      | end
      | 
      | port_label('input', 1, strcat('{}^{world} H_{',prefix,'\_foot}^d'), 'texmode','on');
      | port_label('input', 2, 'Current {}^{world} H_{base}', 'texmode','on')
      | port_label('input', 3, 'Current q_j', 'texmode','on');
      | 
      | 
      | port_label('output', 1, 'Desired {}^{world} H_{base}', 'texmode','on')
      | port_label('output', 2, 'Desired q_j', 'texmode','on');

== system WBToolboxLibrary/wholeBodyStates/Get Estimate ==
  S-Function : S-Function  FunctionName=WBToolbox  Parameters='GetEstimate',robotName,localName,wbiFile,wbiList,estimateType  SFunctionDeploymentMode=off  EnableBusSupport=off
  Estimate : Outport
  wires:
  S-Function/1 -> Estimate/1

== system WBToolboxLibrary/wholeBodyStates/Get Limits ==
  S-Function : S-Function  FunctionName=WBToolbox  Parameters='GetLimits',robotName,localName,wbiFile,wbiList,limitsType  SFunctionDeploymentMode=off  EnableBusSupport=off
  Min : Outport
  Max : Outport  Port=2
  wires:
  S-Function/1 -> Min/1
  S-Function/2 -> Max/1

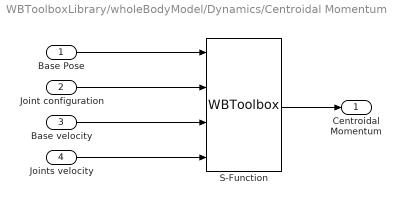
== system WBToolboxLibrary/wholeBodyModel/Dynamics/Centroidal Momentum ==
  Base Pose : Inport
  Joint configuration : Inport  Port=2
  Base velocity : Inport  Port=3
  Joints velocity : Inport  Port=4
  S-Function : S-Function  FunctionName=WBToolbox  Parameters='CentroidalMomentum',robotName,localName,wbiFile,wbiList  SFunctionDeploymentMode=off  EnableBusSupport=off
  Centroidal Momentum : Outport
  wires:
  S-Function/1 -> Centroidal Momentum/1
  Base Pose/1 -> S-Function/1
  Joint configuration/1 -> S-Function/2
  Base velocity/1 -> S-Function/3
  Joints velocity/1 -> S-Function/4

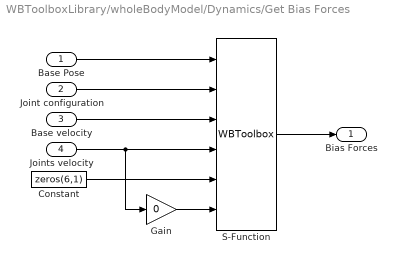
== system WBToolboxLibrary/wholeBodyModel/Dynamics/Get Bias Forces ==
  Base Pose : Inport
  Joint configuration : Inport  Port=2
  Base velocity : Inport  Port=3
  Joints velocity : Inport  Port=4
  Constant : Constant  Value=zeros(6,1)
  Gain : Gain  Gain=0
  S-Function : S-Function  FunctionName=WBToolbox  Parameters='InverseDynamics',robotName,localName,wbiFile,wbiList,explicitGravity  SFunctionDeploymentMode=off  EnableBusSupport=off
  Bias Forces : Outport
  wires:
  S-Function/1 -> Bias Forces/1
  Base Pose/1 -> S-Function/1
  Joint configuration/1 -> S-Function/2
  Base velocity/1 -> S-Function/3
  Joints velocity/1 -> Gain/1, S-Function/4
  Constant/1 -> S-Function/5
  Gain/1 -> S-Function/6

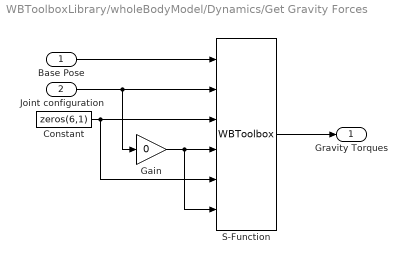
== system WBToolboxLibrary/wholeBodyModel/Dynamics/Get Gravity Forces ==
  Base Pose : Inport
  Joint configuration : Inport  Port=2
  Constant : Constant  Value=zeros(6,1)
  Gain : Gain  Gain=0
  S-Function : S-Function  FunctionName=WBToolbox  Parameters='InverseDynamics',robotName,localName,wbiFile,wbiList,explicitGravity  SFunctionDeploymentMode=off  EnableBusSupport=off
  Gravity Torques : Outport
  wires:
  S-Function/1 -> Gravity Torques/1
  Base Pose/1 -> S-Function/1
  Joint configuration/1 -> Gain/1, S-Function/2
  Constant/1 -> S-Function/5, S-Function/3
  Gain/1 -> S-Function/6, S-Function/4

== system WBToolboxLibrary/wholeBodyModel/Dynamics/Mass Matrix ==
  Base Pose : Inport
  Joint configuration : Inport  Port=2
  S-Function : S-Function  FunctionName=WBToolbox  Parameters='MassMatrix',robotName,localName,wbiFile,wbiList  SFunctionDeploymentMode=off  EnableBusSupport=off
  Mass Matrix : Outport
  wires:
  S-Function/1 -> Mass Matrix/1
  Base Pose/1 -> S-Function/1
  Joint configuration/1 -> S-Function/2
